simulink model "BaseLineCntrl"  (R2016a)
settings: Solver=VariableStepAuto  StartTime=0.0  StopTime=10.0  RelTol=1e-3
values from neighbouring files (symbols this model uses):
  para_cntrl = struct()    [create_para_cntrl_5MWBaseline.m]    (also in para_cntrl_5MWBaseline.mat = )
  para_mdl = struct()    [Regerlung_einer_WEA.m]
settings Model: Creator=leor  LastModifiedBy=leor

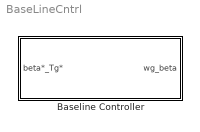
== system BaseLineCntrl ==
  Baseline Controller : Subsystem

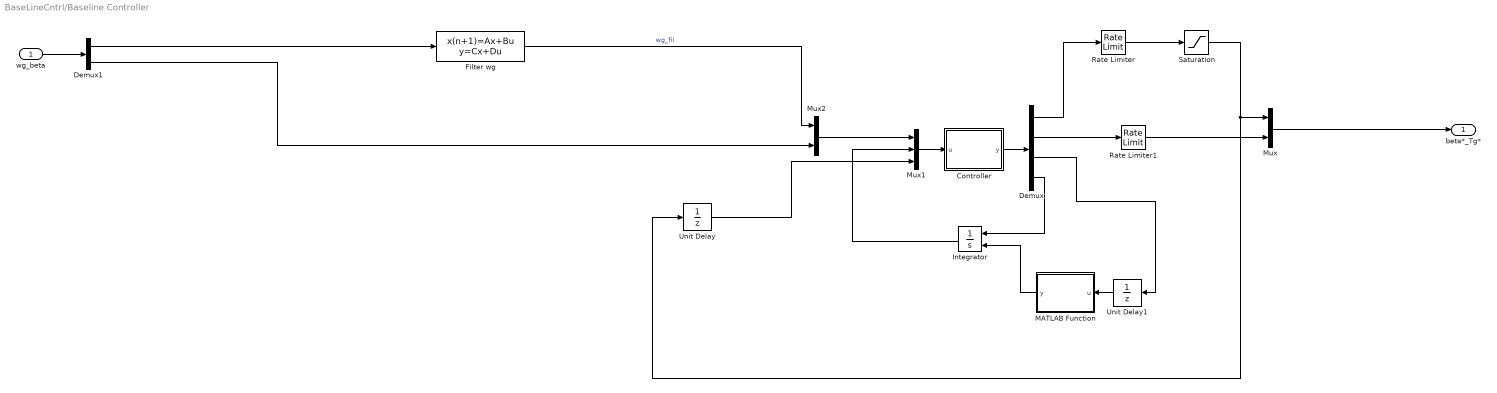
== system BaseLineCntrl/Baseline Controller ==
  wg_beta : Inport
  Controller : MATLAB Function  TreatAsAtomicUnit=on
  Demux : Demux
  Demux1 : Demux  Outputs=2
  Filter wg : DiscreteStateSpace  A=exp(-2*pi*para_mdl.dT*para_cntrl.filter.fc)  B=1-exp(-2*pi*para_mdl.dT*para_cntrl.filter.fc)  C=exp(-2*pi*para_mdl.dT*para_cntrl.filter.fc)  D=1-exp(-2*pi*para_mdl.dT*para_cntrl.filter.fc)  X0=para_cntrl.ref.wg_d  SampleTime=para_mdl.dT
  Integrator : Integrator  ExternalReset=rising  InitialCondition=para_cntrl.initial.int_PCntrl
  MATLAB Function : MATLAB Function  TreatAsAtomicUnit=on
  Mux : Mux  Inputs=2
  Mux1 : Mux  Inputs=3
  Mux2 : Mux  Inputs=2
  Rate Limiter : RateLimiter  RisingSlewLimit=para_cntrl.limits.beta_rate/180*pi  FallingSlewLimit=-para_cntrl.limits.beta_rate/180*pi  SampleTimeMode=inherited
  Rate Limiter1 : RateLimiter  RisingSlewLimit=para_cntrl.limits.Tg_rate  FallingSlewLimit=-para_cntrl.limits.Tg_rate  SampleTimeMode=inherited
  Saturation : Saturate  UpperLimit=90/180*pi  LowerLimit=0
  Unit Delay : UnitDelay  SampleTime=para_mdl.dT
  Unit Delay1 : UnitDelay  SampleTime=para_mdl.dT
  beta*_Tg* : Outport
  wires:
  Rate Limiter1/1 -> Mux/2
  Demux/1 -> Rate Limiter/1
  Mux1/1 -> Controller/1(u)
  Demux/4 -> Integrator/1
  Mux/1 -> beta*_Tg*/1
  Demux/2 -> Rate Limiter1/1
  Controller/1(y) -> Demux/1
  Demux/3 -> Unit Delay1/1
  Integrator/1 -> Mux1/2
  wg_beta/1 -> Demux1/1
  Unit Delay/1 -> Mux1/3
  Demux1/2 -> Mux2/2
  Mux2/1 -> Mux1/1
  Filter wg/1 -> Mux2/1  "wg_fil"
  MATLAB Function/1(y) -> Integrator/2
  Unit Delay1/1 -> MATLAB Function/1(u)
  Rate Limiter/1 -> Saturation/1
  Saturation/1 -> Unit Delay/1, Mux/1
  Demux1/1 -> Filter wg/1

== matlab function BaseLineCntrl/Baseline Controller/MATLAB Function ==
  data: u input; y output
function y = fcn(u)
%#codegen
if u < 5
    y = 1;
else 
    y = 0;
end

== matlab function BaseLineCntrl/Baseline Controller/Controller ==
  data: u input size=4,1; y output; para_cntrl parameter
function y = fcn(u,para_cntrl)
% Regler für den gesamten Arbeitsbereich der Windturbine, für eine
% Beschreibung der Reglerparameter und verwendeten Arbeitspunkte: create_para_cntrl_5MWBaseline.m

% --------------------------------------------------- read inputs
% the input size of u is determined in the simulink model explorer (otherwise Simulink produces errors)

wg = u(1); % in [rad/s]; filtered
beta = u(2)/180*pi; % in [deg]/180*pi = [rad] not used, actually the pitch angle one step before is used for gain scheduling and decision on control region

int_delta_wg = u(3); % integral of the error; used for the pitch controller
beta_prev = u(4);% [rad], previous value of beta_d

% --------------------------------------------------- 

delta_wg = 0;   % set delta_wg to 0 to stop integrating if not in region (3) --> in region 3 delta_wg is defined again

wg_d    = para_cntrl.ref.wg_d;                                 % Solldrehzahl Generator in rad/s
Tgmax   = para_cntrl.ref.Tgmax;                                % max. Generator torque

Kopt =  para_cntrl.Kopt;                                              % Region 2 optimal Torque Open Loop Tg = Kopt*wr^2; kopt from NREL FAST Description
Tg_slope15 = para_cntrl.Tg_slope15;                                   % Region 15, linear ramp from w_cut_in to region 2
Tg_slope25 = para_cntrl.Tg_slope25;%Tgmax/(wg_d-.9*wg_d);
Tgx = para_cntrl.Tgx;

wg_SP_15                  = para_cntrl.ref.wg_SP_15;                    % wg Setpoint for Region 1.5
wg_SP_2                   = para_cntrl.ref.wg_SP_2;                     % wg Setpoint for Region 2
wg_SP_25                  = para_cntrl.ref.wg_SP_25;                    % wg Setpoint for Region 2.5
wg_SP_3                   = para_cntrl.ref.wg_SP_3;                     % wg Setpoint for Region 2.5

% Figure out which Region we are in:                                                                             
if wg < wg_SP_15 && (beta_prev < 1/180*pi) % Region 1
    reg = 1;
elseif wg < wg_SP_2 && (beta_prev < 1/180*pi) % Region 1,5
    reg = 2;
elseif wg < wg_SP_25 && (beta_prev < 1/180*pi) % Region 2
    reg = 3;
elseif (wg < wg_SP_3) && (beta_prev < 1/180*pi)% Region 2,5; NREL 5MW WT Description: 99% of the nominal speed; conditional statement on (beta_prev < 1/180*pi) also from FAST
    reg = 4;
else 
    reg = 5; % Region 3
end

% --------------- set the control output - overwritten in the switch case statement, needed for simulink
uc = [0 ; Tgmax]; 
% ---------------

switch reg 
    case 1 % Region 1
        uc = [0 ; 0];
    case 2 % Region 1.5
        Tg = Tg_slope15 * (wg - wg_SP_15);
        uc = [0 ; Tg];
    case 3 % Region 2
        Tg = Kopt*(wg*30/pi)^2; % Kopt is in [Nm/rpm^2]
        uc = [0 ; Tg];
    case 4 % Region 2.5
        Tg = Tg_slope25*wg + Tgx; % Tg_slope25 in [Nm/rad/s]
        if Tg > Tgmax
            disp(Tg-Tgmax)
            Tg = Tgmax;
        end
        uc = [0 ; Tg];
    case 5 % Region 3
        
        % calculation of the Pitch Angle
        betak = para_cntrl.ref.betak;    % in combination with beta_previous determines the scheduling
        Kp = para_cntrl.Kp0*1/(1+beta_prev/betak);
        Ki = para_cntrl.Ki0*1/(1+beta_prev/betak);
        delta_wg = (wg-wg_d);
        betad = (Kp*delta_wg + Ki*int_delta_wg); % in [rad]
        
        %calculation of the torque
        if wg < wg_d 
            Tg = Tg_slope25*wg + Tgx;
            if Tg < (Tg_slope25*.99*wg_d + Tgx)
                Tg = Tg_slope25*.99*wg_d + Tgx;
            end
        elseif para_cntrl.var_Trq_Reg3 == 1 
            Tg = para_cntrl.para.P0/wg;
        else
            Tg = Tgmax;
        end
        uc = [betad ; Tg]; 
end
y = [uc ; reg ; delta_wg];
